simulink model "MSD"  (R2020a)
settings: Solver=VariableStepAuto  StartTime=0.0  StopTime=10.0  RelTol=1e-3
values from neighbouring files (symbols this model uses):
  A = [0 1; -k/m -c/m]    [param_MSD.m]
  B = [0; 1/m]    [param_MSD.m]
  K = place(A,B,P)    [param_MSD.m]
settings Model: Creator=fukao  LastModifiedBy=fukao
settings DebuggingCC: SFMachineParentedDataDiag=error

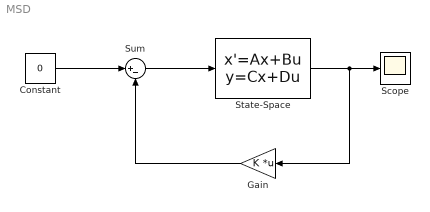
== system MSD ==
  Constant : Constant  Value=0
  Gain : Gain  Gain=K  Multiplication=Matrix(K*u)
  Scope : Scope
  State-Space : StateSpace  A=A  B=B  C=eye(2)  D=zeros(2,1)  InitialCondition=[1 ; 0]
  Sum : Sum  Inputs=|+-
  wires:
  Constant/1 -> Sum/1
  Sum/1 -> State-Space/1
  State-Space/1 -> Gain/1, Scope/1
  Gain/1 -> Sum/2
